simulink model "line_CF1_FS"  (R2018b)
settings: Solver=FixedStepAuto  StartTime=0.0  StopTime=inf  FixedStep=0.01  RelTol=1e-3
undefined symbols (not defined in the file or in its folder): Angular, Linear
libraries: autolibshared x10, vehdynlibsteering x10, robotlib x7, peGeneralControl x1
(part 2 of 2)

== system line_CF1_FS/Human Follower 4/Reaction Time ==
  v_new : Inport
  v_old : Inport  Port=2
  Delay : Delay  DelayLength=3  InitialConditionSource=Input port
      settings: InputPortMap=u0,p4
  If Action Subsystem3 : Subsystem  TreatAsAtomicUnit=on
  If Action Subsystem5 : Subsystem  TreatAsAtomicUnit=on
  If2 : If  NumInputs=2  IfExpression=u2 ~= u1
  Merge1 : Merge
  v_out : Outport
  wires:
  If Action Subsystem5/1(Out1) -> Merge1/2
  If2/1 -> If Action Subsystem3/Action
  If2/2 -> If Action Subsystem5/Action
  If Action Subsystem3/1(Out1) -> Merge1/1
  v_new/1 -> If2/1, If Action Subsystem3/1(In1)
  Merge1/1 -> Delay/1
  Delay/1 -> v_out/1
  v_old/1 -> If2/2, Delay/2, If Action Subsystem5/1(In1)

== system line_CF1_FS/Human Follower 5/Human Follower model ==
  note: relitive distance
  note: relitive velocity
  this cars vel : Inport
  lead cars vel_x : Inport  Port=2
  max vel : Inport  Port=3
  lead cars dist_x : Inport  Port=4
  this cars dist_x : Inport  Port=5
  sampling time : Inport  Port=6
  Add : Sum
  Human Follower math : Subsystem
  Multiply : Product
  Subtract2 : Sum  Inputs=+-
  Subtract3 : Sum  Inputs=+-
  cmd Vel : Outport
  wires:
  Add/1 -> cmd Vel/1
  lead cars dist_x/1 -> Subtract3/1
  this cars vel/1 -> Human Follower math/3(v), Add/1, Subtract2/2
  Human Follower math/1(a_cmd) -> Multiply/2
  Subtract3/1 -> Human Follower math/2(dx)
  Multiply/1 -> Add/2
  this cars dist_x/1 -> Subtract3/2
  Subtract2/1 -> Human Follower math/1(dv)
  max vel/1 -> Human Follower math/4(v_max)
  sampling time/1 -> Multiply/1
  lead cars vel_x/1 -> Subtract2/1

== system line_CF1_FS/Human Follower 5/Reaction Time ==
  v_new : Inport
  v_old : Inport  Port=2
  Delay : Delay  DelayLength=3  InitialConditionSource=Input port
      settings: InputPortMap=u0,p4
  If Action Subsystem3 : Subsystem  TreatAsAtomicUnit=on
  If Action Subsystem5 : Subsystem  TreatAsAtomicUnit=on
  If2 : If  NumInputs=2  IfExpression=u2 ~= u1
  Merge1 : Merge
  v_out : Outport
  wires:
  If Action Subsystem5/1(Out1) -> Merge1/2
  If2/1 -> If Action Subsystem3/Action
  If2/2 -> If Action Subsystem5/Action
  If Action Subsystem3/1(Out1) -> Merge1/1
  v_new/1 -> If2/1, If Action Subsystem3/1(In1)
  Merge1/1 -> Delay/1
  Delay/1 -> v_out/1
  v_old/1 -> If2/2, Delay/2, If Action Subsystem5/1(In1)

== system line_CF1_FS/Human Follower 6/Human Follower model ==
  note: relitive distance
  note: relitive velocity
  this cars vel : Inport
  lead cars vel_x : Inport  Port=2
  max vel : Inport  Port=3
  lead cars dist_x : Inport  Port=4
  this cars dist_x : Inport  Port=5
  sampling time : Inport  Port=6
  Add : Sum
  Human Follower math : Subsystem
  Multiply : Product
  Subtract2 : Sum  Inputs=+-
  Subtract3 : Sum  Inputs=+-
  cmd Vel : Outport
  wires:
  Add/1 -> cmd Vel/1
  lead cars dist_x/1 -> Subtract3/1
  this cars vel/1 -> Human Follower math/3(v), Add/1, Subtract2/2
  Human Follower math/1(a_cmd) -> Multiply/2
  Subtract3/1 -> Human Follower math/2(dx)
  Multiply/1 -> Add/2
  this cars dist_x/1 -> Subtract3/2
  Subtract2/1 -> Human Follower math/1(dv)
  max vel/1 -> Human Follower math/4(v_max)
  sampling time/1 -> Multiply/1
  lead cars vel_x/1 -> Subtract2/1

== system line_CF1_FS/Human Follower 6/Reaction Time ==
  v_new : Inport
  v_old : Inport  Port=2
  Delay : Delay  DelayLength=3  InitialConditionSource=Input port
      settings: InputPortMap=u0,p4
  If Action Subsystem3 : Subsystem  TreatAsAtomicUnit=on
  If Action Subsystem5 : Subsystem  TreatAsAtomicUnit=on
  If2 : If  NumInputs=2  IfExpression=u2 ~= u1
  Merge1 : Merge
  v_out : Outport
  wires:
  If Action Subsystem5/1(Out1) -> Merge1/2
  If2/1 -> If Action Subsystem3/Action
  If2/2 -> If Action Subsystem5/Action
  If Action Subsystem3/1(Out1) -> Merge1/1
  v_new/1 -> If2/1, If Action Subsystem3/1(In1)
  Merge1/1 -> Delay/1
  Delay/1 -> v_out/1
  v_old/1 -> If2/2, Delay/2, If Action Subsystem5/1(In1)

== system line_CF1_FS/Human Follower 7/Human Follower model ==
  note: relitive distance
  note: relitive velocity
  this cars vel : Inport
  lead cars vel_x : Inport  Port=2
  max vel : Inport  Port=3
  lead cars dist_x : Inport  Port=4
  this cars dist_x : Inport  Port=5
  sampling time : Inport  Port=6
  Add : Sum
  Human Follower math : Subsystem
  Multiply : Product
  Subtract2 : Sum  Inputs=+-
  Subtract3 : Sum  Inputs=+-
  cmd Vel : Outport
  wires:
  Add/1 -> cmd Vel/1
  lead cars dist_x/1 -> Subtract3/1
  this cars vel/1 -> Human Follower math/3(v), Add/1, Subtract2/2
  Human Follower math/1(a_cmd) -> Multiply/2
  Subtract3/1 -> Human Follower math/2(dx)
  Multiply/1 -> Add/2
  this cars dist_x/1 -> Subtract3/2
  Subtract2/1 -> Human Follower math/1(dv)
  max vel/1 -> Human Follower math/4(v_max)
  sampling time/1 -> Multiply/1
  lead cars vel_x/1 -> Subtract2/1

== system line_CF1_FS/Human Follower 7/Reaction Time ==
  v_new : Inport
  v_old : Inport  Port=2
  Delay : Delay  DelayLength=3  InitialConditionSource=Input port
      settings: InputPortMap=u0,p4
  If Action Subsystem3 : Subsystem  TreatAsAtomicUnit=on
  If Action Subsystem5 : Subsystem  TreatAsAtomicUnit=on
  If2 : If  NumInputs=2  IfExpression=u2 ~= u1
  Merge1 : Merge
  v_out : Outport
  wires:
  If Action Subsystem5/1(Out1) -> Merge1/2
  If2/1 -> If Action Subsystem3/Action
  If2/2 -> If Action Subsystem5/Action
  If Action Subsystem3/1(Out1) -> Merge1/1
  v_new/1 -> If2/1, If Action Subsystem3/1(In1)
  Merge1/1 -> Delay/1
  Delay/1 -> v_out/1
  v_old/1 -> If2/2, Delay/2, If Action Subsystem5/1(In1)

== system line_CF1_FS/Human Follower 8/Human Follower model ==
  note: relitive distance
  note: relitive velocity
  this cars vel : Inport
  lead cars vel_x : Inport  Port=2
  max vel : Inport  Port=3
  lead cars dist_x : Inport  Port=4
  this cars dist_x : Inport  Port=5
  sampling time : Inport  Port=6
  Add : Sum
  Human Follower math : Subsystem
  Multiply : Product
  Subtract2 : Sum  Inputs=+-
  Subtract3 : Sum  Inputs=+-
  cmd Vel : Outport
  wires:
  Add/1 -> cmd Vel/1
  lead cars dist_x/1 -> Subtract3/1
  this cars vel/1 -> Human Follower math/3(v), Add/1, Subtract2/2
  Human Follower math/1(a_cmd) -> Multiply/2
  Subtract3/1 -> Human Follower math/2(dx)
  Multiply/1 -> Add/2
  this cars dist_x/1 -> Subtract3/2
  Subtract2/1 -> Human Follower math/1(dv)
  max vel/1 -> Human Follower math/4(v_max)
  sampling time/1 -> Multiply/1
  lead cars vel_x/1 -> Subtract2/1

== system line_CF1_FS/Human Follower 8/Reaction Time ==
  v_new : Inport
  v_old : Inport  Port=2
  Delay : Delay  DelayLength=3  InitialConditionSource=Input port
      settings: InputPortMap=u0,p4
  If Action Subsystem3 : Subsystem  TreatAsAtomicUnit=on
  If Action Subsystem5 : Subsystem  TreatAsAtomicUnit=on
  If2 : If  NumInputs=2  IfExpression=u2 ~= u1
  Merge1 : Merge
  v_out : Outport
  wires:
  If Action Subsystem5/1(Out1) -> Merge1/2
  If2/1 -> If Action Subsystem3/Action
  If2/2 -> If Action Subsystem5/Action
  If Action Subsystem3/1(Out1) -> Merge1/1
  v_new/1 -> If2/1, If Action Subsystem3/1(In1)
  Merge1/1 -> Delay/1
  Delay/1 -> v_out/1
  v_old/1 -> If2/2, Delay/2, If Action Subsystem5/1(In1)

== system line_CF1_FS/Human Follower 1/Human Follower model/Human Follower math ==
  dv : Inport
  dx : Inport  Port=2
  v : Inport  Port=3
  v_max : Inport  Port=4
  MATLAB Function : MATLAB Function  TreatAsAtomicUnit=on
  a_cmd : Outport
  wires:
  v_max/1 -> MATLAB Function/4(v_max)
  MATLAB Function/1(acceleration) -> a_cmd/1
  v/1 -> MATLAB Function/3(v)
  dv/1 -> MATLAB Function/1(dv)
  dx/1 -> MATLAB Function/2(dx)

== system line_CF1_FS/Human Follower 1/Reaction Time/If Action Subsystem3 ==
  In1 : Inport
  Action Port : ActionPort  ActionType=then
  Out1 : Outport
  wires:
  In1/1 -> Out1/1

== system line_CF1_FS/Human Follower 1/Reaction Time/If Action Subsystem5 ==
  In1 : Inport
  Action Port : ActionPort  ActionType=else
  Out1 : Outport
  wires:
  In1/1 -> Out1/1

== system line_CF1_FS/Human Follower 2/Human Follower model/Human Follower math ==
  dv : Inport
  dx : Inport  Port=2
  v : Inport  Port=3
  v_max : Inport  Port=4
  MATLAB Function : MATLAB Function  TreatAsAtomicUnit=on
  a_cmd : Outport
  wires:
  v_max/1 -> MATLAB Function/4(v_max)
  MATLAB Function/1(acceleration) -> a_cmd/1
  v/1 -> MATLAB Function/3(v)
  dv/1 -> MATLAB Function/1(dv)
  dx/1 -> MATLAB Function/2(dx)

== system line_CF1_FS/Human Follower 2/Reaction Time/If Action Subsystem3 ==
  In1 : Inport
  Action Port : ActionPort  ActionType=then
  Out1 : Outport
  wires:
  In1/1 -> Out1/1

== system line_CF1_FS/Human Follower 2/Reaction Time/If Action Subsystem5 ==
  In1 : Inport
  Action Port : ActionPort  ActionType=else
  Out1 : Outport
  wires:
  In1/1 -> Out1/1

== system line_CF1_FS/Human Follower 3/Human Follower model/Human Follower math ==
  dv : Inport
  dx : Inport  Port=2
  v : Inport  Port=3
  v_max : Inport  Port=4
  MATLAB Function : MATLAB Function  TreatAsAtomicUnit=on
  a_cmd : Outport
  wires:
  v_max/1 -> MATLAB Function/4(v_max)
  MATLAB Function/1(acceleration) -> a_cmd/1
  v/1 -> MATLAB Function/3(v)
  dv/1 -> MATLAB Function/1(dv)
  dx/1 -> MATLAB Function/2(dx)

== system line_CF1_FS/Human Follower 3/Reaction Time/If Action Subsystem3 ==
  In1 : Inport
  Action Port : ActionPort  ActionType=then
  Out1 : Outport
  wires:
  In1/1 -> Out1/1

== system line_CF1_FS/Human Follower 3/Reaction Time/If Action Subsystem5 ==
  In1 : Inport
  Action Port : ActionPort  ActionType=else
  Out1 : Outport
  wires:
  In1/1 -> Out1/1

== system line_CF1_FS/Human Follower 4/Human Follower model/Human Follower math ==
  dv : Inport
  dx : Inport  Port=2
  v : Inport  Port=3
  v_max : Inport  Port=4
  MATLAB Function : MATLAB Function  TreatAsAtomicUnit=on
  a_cmd : Outport
  wires:
  v_max/1 -> MATLAB Function/4(v_max)
  MATLAB Function/1(acceleration) -> a_cmd/1
  v/1 -> MATLAB Function/3(v)
  dv/1 -> MATLAB Function/1(dv)
  dx/1 -> MATLAB Function/2(dx)

== system line_CF1_FS/Human Follower 4/Reaction Time/If Action Subsystem3 ==
  In1 : Inport
  Action Port : ActionPort  ActionType=then
  Out1 : Outport
  wires:
  In1/1 -> Out1/1

== system line_CF1_FS/Human Follower 4/Reaction Time/If Action Subsystem5 ==
  In1 : Inport
  Action Port : ActionPort  ActionType=else
  Out1 : Outport
  wires:
  In1/1 -> Out1/1

== system line_CF1_FS/Human Follower 5/Human Follower model/Human Follower math ==
  dv : Inport
  dx : Inport  Port=2
  v : Inport  Port=3
  v_max : Inport  Port=4
  MATLAB Function : MATLAB Function  TreatAsAtomicUnit=on
  a_cmd : Outport
  wires:
  v_max/1 -> MATLAB Function/4(v_max)
  MATLAB Function/1(acceleration) -> a_cmd/1
  v/1 -> MATLAB Function/3(v)
  dv/1 -> MATLAB Function/1(dv)
  dx/1 -> MATLAB Function/2(dx)

== system line_CF1_FS/Human Follower 5/Reaction Time/If Action Subsystem3 ==
  In1 : Inport
  Action Port : ActionPort  ActionType=then
  Out1 : Outport
  wires:
  In1/1 -> Out1/1

== system line_CF1_FS/Human Follower 5/Reaction Time/If Action Subsystem5 ==
  In1 : Inport
  Action Port : ActionPort  ActionType=else
  Out1 : Outport
  wires:
  In1/1 -> Out1/1

== system line_CF1_FS/Human Follower 6/Human Follower model/Human Follower math ==
  dv : Inport
  dx : Inport  Port=2
  v : Inport  Port=3
  v_max : Inport  Port=4
  MATLAB Function : MATLAB Function  TreatAsAtomicUnit=on
  a_cmd : Outport
  wires:
  v_max/1 -> MATLAB Function/4(v_max)
  MATLAB Function/1(acceleration) -> a_cmd/1
  v/1 -> MATLAB Function/3(v)
  dv/1 -> MATLAB Function/1(dv)
  dx/1 -> MATLAB Function/2(dx)

== system line_CF1_FS/Human Follower 6/Reaction Time/If Action Subsystem3 ==
  In1 : Inport
  Action Port : ActionPort  ActionType=then
  Out1 : Outport
  wires:
  In1/1 -> Out1/1

== system line_CF1_FS/Human Follower 6/Reaction Time/If Action Subsystem5 ==
  In1 : Inport
  Action Port : ActionPort  ActionType=else
  Out1 : Outport
  wires:
  In1/1 -> Out1/1

== system line_CF1_FS/Human Follower 7/Human Follower model/Human Follower math ==
  dv : Inport
  dx : Inport  Port=2
  v : Inport  Port=3
  v_max : Inport  Port=4
  MATLAB Function : MATLAB Function  TreatAsAtomicUnit=on
  a_cmd : Outport
  wires:
  v_max/1 -> MATLAB Function/4(v_max)
  MATLAB Function/1(acceleration) -> a_cmd/1
  v/1 -> MATLAB Function/3(v)
  dv/1 -> MATLAB Function/1(dv)
  dx/1 -> MATLAB Function/2(dx)

== system line_CF1_FS/Human Follower 7/Reaction Time/If Action Subsystem3 ==
  In1 : Inport
  Action Port : ActionPort  ActionType=then
  Out1 : Outport
  wires:
  In1/1 -> Out1/1

== system line_CF1_FS/Human Follower 7/Reaction Time/If Action Subsystem5 ==
  In1 : Inport
  Action Port : ActionPort  ActionType=else
  Out1 : Outport
  wires:
  In1/1 -> Out1/1

== system line_CF1_FS/Human Follower 8/Human Follower model/Human Follower math ==
  dv : Inport
  dx : Inport  Port=2
  v : Inport  Port=3
  v_max : Inport  Port=4
  MATLAB Function : MATLAB Function  TreatAsAtomicUnit=on
  a_cmd : Outport
  wires:
  v_max/1 -> MATLAB Function/4(v_max)
  MATLAB Function/1(acceleration) -> a_cmd/1
  v/1 -> MATLAB Function/3(v)
  dv/1 -> MATLAB Function/1(dv)
  dx/1 -> MATLAB Function/2(dx)

== system line_CF1_FS/Human Follower 8/Reaction Time/If Action Subsystem3 ==
  In1 : Inport
  Action Port : ActionPort  ActionType=then
  Out1 : Outport
  wires:
  In1/1 -> Out1/1

== system line_CF1_FS/Human Follower 8/Reaction Time/If Action Subsystem5 ==
  In1 : Inport
  Action Port : ActionPort  ActionType=else
  Out1 : Outport
  wires:
  In1/1 -> Out1/1

== matlab function line_CF1_FS/FollowerStopper Controller/Dead Man's Switch/timeout set to 0 output ==
  data: isNew input; safeValue output; value input; timeout input; timedOut output; stepSize input
function [safeValue,timedOut] = fcn(isNew,value,timeout,stepSize)
%#codegen
persistent sinceLastMsg
timedOut=true;
if isempty(sinceLastMsg)
    sinceLastMsg=(timeout/stepSize)+1;
end

safeValue=0;
% if no new message
% after timeout, we output 0
if( isNew == true )
    sinceLastMsg = 0;
else
    sinceLastMsg = sinceLastMsg+1;
end

% Note: we require step size as an input here, and depend on our
% system being executed at a regular rate, or bad things will happen
if( sinceLastMsg < timeout/stepSize )
    timedOut = false;
end
    
if( timedOut == false )
    safeValue = value;
end

== matlab function line_CF1_FS/FollowerStopper Controller/MATLAB Function ==
  settings: updateMethod=DISCRETE
  data: max_speed input; u_out output; vel input; max_accel input; max_decel input
function u_out = fcn(max_speed,vel,max_accel,max_decel)
% #codegen
persistent y

if isempty(y)
    y=vel;
end

dt=0.01;
if( y > max_speed + max_accel*dt)
    y = max(max_speed,y - abs(max_decel)*dt);
elseif( y < max_speed - abs(max_decel)*dt)
    y = min(max_speed,y + max_accel*dt);
else
    y = max_speed;
end

u_out = y;

== matlab function line_CF1_FS/Human Follower 2/Human Follower model/Human Follower math/MATLAB Function ==
  data: dv input; dx input; v input; v_max input; acceleration output
function acceleration = fcn(dv, dx, v, v_max)

sd = 2;

if v + dv < 0
    V = 0;
end

if dx <= sd
    V = 0;
elseif dx <= 35
    V = dx - (5 + sd);
else
    V = 30;
end

if dv + v <= v_max
    w = v + dv;
else
    w = v_max;
end

acceleration = 0.1*(V-v) + 0.5*(w-v);

== matlab function line_CF1_FS/Human Follower 3/Human Follower model/Human Follower math/MATLAB Function ==
  data: dv input; dx input; v input; v_max input; acceleration output
function acceleration = fcn(dv, dx, v, v_max)

sd = 2;

if v + dv < 0
    V = 0;
end

if dx <= sd
    V = 0;
elseif dx <= 35
    V = dx - (5 + sd);
else
    V = 30;
end

if dv + v <= v_max
    w = v + dv;
else
    w = v_max;
end

acceleration = 0.1*(V-v) + 0.5*(w-v);

== matlab function line_CF1_FS/Human Follower 1/Human Follower model/Human Follower math/MATLAB Function ==
  data: dv input; dx input; v input; v_max input; acceleration output
function acceleration = fcn(dv, dx, v, v_max)
sd = 2;

if v + dv < 0
    V = 0;
end
if dx <= sd
    V = 0;
elseif dx <= 35
    V = dx - (5 + sd);
else
    V = 30;
end

if dv + v <= v_max
    w = v + dv;
else
    w = v_max;
end

acceleration = 0.1*(V-v) + 0.5*(w-v);

== matlab function line_CF1_FS/FollowerStopper Controller/Follower Stopper Controller/MATLAB Function ==
  data: r input; u_cmd output; dx input; dv input; v_AV input; dx_min input; dx_activate input; decel input
function u_cmd = fcn(r,dx,dv,v_AV,...
    dx_min,dx_activate,decel)
%#codegen
% Safety controller, based on quadratic bands.
% Input: r = desired velocity (from other models)
%          dx = estimate of gap to vehicle ahead
%          dv = estimate of time derivative of dx (= velocity difference)
%         v_AV = velocity of AV
%      dx_min = minimum distance
% dx_activate = distance below which controller does something
%       decel = vector of three deceleration values for parabolas
% Out:  u_cmd = actual velocity commanded (always u_cmd<=U)
%
% Controller-specific parameters
dx_mid = (dx_min+dx_activate)/2; % mid distance, where v_lead is commanded
% Lead vehicle velocity
v_lead = v_AV+dv; % velocity of lead vehicle
v_lead = max(v_lead,0); % lead vehicle cannot go backwards
v = min(r,v_lead); % safety velocity cannot exceed desired velocity U
% Treatment of positive dv-values
dv = min(dv,0); % domains for dv>0 same as dv=0
% For given dv, dx-values of band boundaries
dx1 = dx_min+1/(2*decel(1))*dv.^2;
dx2 = dx_mid+1/(2*decel(2))*dv.^2;
dx3 = dx_activate+1/(2*decel(3))*dv.^2;

% Actual commanded velocity
dt = 0.01;
max_accel = 1.5;
smoothChange = v_AV + max_accel*dt;
if (dx <= dx1)
    u_cmd = 0;
elseif (dx <= dx2)
    u_cmd = min(v*(dx-dx1)/(dx2-dx1) , smoothChange);
elseif (dx <= dx3)
    u_cmd = min(v + (r-v)*(dx-dx2)/(dx3-dx2) , smoothChange);
else
    u_cmd = min(r , smoothChange);
end

== matlab function line_CF1_FS/Human Follower 4/Human Follower model/Human Follower math/MATLAB Function ==
  data: dv input; dx input; v input; v_max input; acceleration output
function acceleration = fcn(dv, dx, v, v_max)

sd = 2;

if v + dv < 0
    V = 0;
end

if dx <= sd
    V = 0;
elseif dx <= 35
    V = dx - (5 + sd);
else
    V = 30;
end

if dv + v <= v_max
    w = v + dv;
else
    w = v_max;
end

acceleration = 0.1*(V-v) + 0.5*(w-v);

== matlab function line_CF1_FS/Human Follower 5/Human Follower model/Human Follower math/MATLAB Function ==
  data: dv input; dx input; v input; v_max input; acceleration output
function acceleration = fcn(dv, dx, v, v_max)

sd = 2;

if v + dv < 0
    V = 0;
end

if dx <= sd
    V = 0;
elseif dx <= 35
    V = dx - (5 + sd);
else
    V = 30;
end

if dv + v <= v_max
    w = v + dv;
else
    w = v_max;
end

acceleration = 0.1*(V-v) + 0.5*(w-v);

== matlab function line_CF1_FS/Human Follower 6/Human Follower model/Human Follower math/MATLAB Function ==
  data: dv input; dx input; v input; v_max input; acceleration output
function acceleration = fcn(dv, dx, v, v_max)

sd = 2;

if v + dv < 0
    V = 0;
end

if dx <= sd
    V = 0;
elseif dx <= 35
    V = dx - (5 + sd);
else
    V = 30;
end

if dv + v <= v_max
    w = v + dv;
else
    w = v_max;
end

acceleration = 0.1*(V-v) + 0.5*(w-v);

== matlab function line_CF1_FS/Human Follower 7/Human Follower model/Human Follower math/MATLAB Function ==
  data: dv input; dx input; v input; v_max input; acceleration output
function acceleration = fcn(dv, dx, v, v_max)

sd = 2;

if v + dv < 0
    V = 0;
end

if dx <= sd
    V = 0;
elseif dx <= 35
    V = dx - (5 + sd);
else
    V = 30;
end

if dv + v <= v_max
    w = v + dv;
else
    w = v_max;
end

acceleration = 0.1*(V-v) + 0.5*(w-v);

== matlab function line_CF1_FS/Human Follower 8/Human Follower model/Human Follower math/MATLAB Function ==
  data: dv input; dx input; v input; v_max input; acceleration output
function acceleration = fcn(dv, dx, v, v_max)

sd = 2;

if v + dv < 0
    V = 0;
end

if dx <= sd
    V = 0;
elseif dx <= 35
    V = dx - (5 + sd);
else
    V = 30;
end

if dv + v <= v_max
    w = v + dv;
else
    w = v_max;
end

acceleration = 0.1*(V-v) + 0.5*(w-v);
